simulink model "GlideslopeController_model"  (R2020b)
settings: Solver=VariableStepAuto  StartTime=0.0  StopTime=2000  RelTol=1e-3
values from neighbouring files (symbols this model uses):
  A_red_lo = sel(A_longitude_lo, [1 3 4 2 5], [1 3 4 2 5])    [GlideslopeController.m]
  B_red_lo = sel(A_longitude_lo, [1 3 4 2 5], [6 7])    [GlideslopeController.m]
  C_red_lo = sel(C_longitude_lo, [1 3 4 2 5], [1 3 4 2 5])    [GlideslopeController.m]
  D_red_lo = sel(C_longitude_lo, [1 3 4 2 5], [6 7])    [GlideslopeController.m]
  Kglide = 50    [GlideslopeController.m]
  Kq = -1    [GlideslopeController.m]
  Ktheta = 2    [GlideslopeController.m]
  Kv = 500    [GlideslopeController.m]
undefined symbols (not defined in the file or in its folder): magnitude, trim_control_lo, trim_state_lo, trim_thrust_lo
libraries: simulink_extras x10, simulink x1
settings Model: Creator=viran  LastModifiedBy=viran

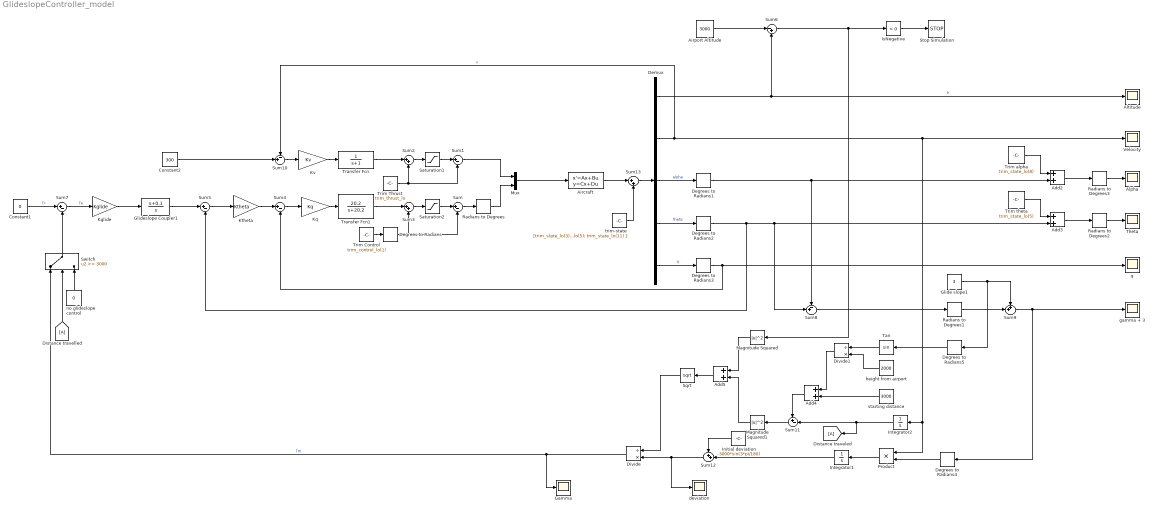
== system GlideslopeController_model ==
  " Glideslope Coupler1" : TransferFcn  Numerator=[1 0.1]  Denominator=[1 0]
  Add{2..5} (4 alike) : Sum
  Aircraft : StateSpace  A=A_red_lo  B=B_red_lo  C=C_red_lo  D=D_red_lo  InitialCondition=0
  Airport Altitude : Constant  Value=3000
  Alpha : Scope
  Altitude : Scope
  Constant1 : Constant  Value=0
  Constant2 : Constant  Value=300
  Degrees to Radians{,1..5} (6 alike) : simulink_extras/Transformations/Degrees to Radians
  Demux : Demux  Outputs=5
  Divide : Product  Inputs=/*
  Divide1 : Product  Inputs=/*
  Gamma : Scope
  Glide slope1 : Constant  Value=3
  Initial deviation : Constant  Value=-3000*sin(3*pi/180)
  Integrator1 : Integrator
  Integrator2 : Integrator
  IsNegative : simulink/Logic and Bit Operations/Compare To Zero  relop=<  OutDataTypeStr=boolean
  Kglide : Gain  Gain=Kglide
  Kq : Gain  Gain=Kq
  Ktheta : Gain  Gain=Ktheta
  Kv : Gain  Gain=Kv
  Magnitude Squared : Math  Operator=magnitude^2  SaturateOnIntegerOverflow=on
  Magnitude Squared1 : Math  Operator=magnitude^2  SaturateOnIntegerOverflow=on
  Mux : Mux  Inputs=2
  Product : Product
  Radians to Degrees{,1..3} (4 alike) : simulink_extras/Transformations/Radians to Degrees
  Saturation1 : Saturate  UpperLimit=19000  LowerLimit=1000
  Saturation2 : Saturate  UpperLimit=25*pi/180  LowerLimit=-25*pi/180
  Sqrt : Sqrt  SaturateOnIntegerOverflow=on
  Stop Simulation : Stop
  Sum{,1,4..5,7} (5 alike) : Sum  Inputs=|+-
  Sum10 : Sum  Inputs=-+|
  Sum11 : Sum  Inputs=+-|
  Sum12 : Sum  Inputs=++|
  Sum13 : Sum  Inputs=|++
  Sum2 : Sum  Inputs=|++
  Sum3 : Sum  Inputs=|++
  Sum6 : Sum  Inputs=|-+
  Sum8 : Sum  Inputs=-+|
  Sum9 : Sum  Inputs=++|
  Switch : Switch  Threshold=3000
  Tan : Trigonometry
  Theta : Scope
  Transfer Fcn : TransferFcn  Denominator=[1 1]
  Transfer Fcn1 : TransferFcn  Numerator=[20.2]  Denominator=[1 20.2]
  Trim Control : Constant  Value=trim_control_lo(1)
  Trim Thrust : Constant  Value=trim_thrust_lo
  Trim alpha : Constant  Value=trim_state_lo(8)
  Trim theta : Constant  Value=trim_state_lo(5)
  Velocity : Scope
  deviation : Scope
  gamma + 3 : Scope
  height from airport : Constant  Value=2000
  no glideslope control : Constant  Value=0
  q : Scope
  starting distance : Constant  Value=3000
  trim-state : Constant  Value=[trim_state_lo(3); trim_state_lo(7); trim_state_lo(8); trim_state_lo(5); trim_state_lo(11) ]
  wires:
  Mux/1 -> Aircraft/1
  Sum1/1 -> Mux/1
  Aircraft/1 -> Sum13/1
  Demux/3 -> Degrees to Radians1/1  "alpha"
  Demux/4 -> Degrees to Radians2/1  "theta"
  Demux/5 -> Degrees to Radians3/1  "q"
  Saturation1/1 -> Sum1/1
  Saturation2/1 -> Sum/1
  Trim Thrust/1 -> Sum1/2, Sum2/2
  Sum3/1 -> Saturation2/1
  Transfer Fcn1/1 -> Sum3/1
  Sum2/1 -> Saturation1/1
  Transfer Fcn/1 -> Sum2/1
  Trim Control/1 -> Degrees to Radians/1
  Degrees to Radians/1 -> Sum/2, Sum3/2
  Sum/1 -> Radians to Degrees/1
  Radians to Degrees/1 -> Mux/2
  Kv/1 -> Transfer Fcn/1
  Demux/1 -> Sum6/2, Altitude/1  "h"
  Demux/2 -> Sum10/1, Velocity/1, Product/1, Integrator2/1  "v"
  Sum4/1 -> Kq/1
  Kq/1 -> Transfer Fcn1/1
  Ktheta/1 -> Sum4/1
  Sum5/1 -> Ktheta/1
  " Glideslope Coupler1"/1 -> Sum5/1
  Sum10/1 -> Kv/1
  Constant2/1 -> Sum10/2
  Airport Altitude/1 -> Sum6/1
  Sum6/1 -> Magnitude Squared/1, IsNegative/1
  IsNegative/1 -> Stop Simulation/1
  Degrees to Radians1/1 -> Sum8/1, Add2/2
  Degrees to Radians2/1 -> Sum8/2, Add3/2, Sum5/2
  Add2/1 -> Radians to Degrees3/1
  Add3/1 -> Radians to Degrees2/1
  Degrees to Radians3/1 -> q/1, Sum4/2
  Trim alpha/1 -> Add2/1
  Trim theta/1 -> Add3/1
  Kglide/1 -> " Glideslope Coupler1"/1
  Sum7/1 -> Kglide/1  "Γe"
  Constant1/1 -> Sum7/1  "Γr"
  Radians to Degrees2/1 -> Theta/1
  Radians to Degrees3/1 -> Alpha/1
  Sum8/1 -> Radians to Degrees1/1
  Radians to Degrees1/1 -> Sum9/2
  Sum9/1 -> Degrees to Radians4/1, gamma + 3/1
  Glide slope1/1 -> Degrees to Radians5/1, Sum9/1
  Degrees to Radians4/1 -> Product/2
  Product/1 -> Integrator1/1
  Integrator1/1 -> Sum12/2
  no glideslope control/1 -> Switch/3
  Integrator2/1 -> [A], Sum11/2
  Sum11/1 -> Magnitude Squared1/1
  Degrees to Radians5/1 -> Tan/1
  height from airport/1 -> Divide1/2
  Tan/1 -> Divide1/1
  Add4/1 -> Sum11/1
  Divide1/1 -> Add4/1
  starting distance/1 -> Add4/2
  Magnitude Squared/1 -> Add5/1
  Magnitude Squared1/1 -> Add5/2
  Add5/1 -> Sqrt/1
  Sqrt/1 -> Divide/1
  Divide/1 -> Switch/1, Gamma/1  "Γm"
  Sum12/1 -> deviation/1, Divide/2
  Initial deviation/1 -> Sum12/1
  Sum13/1 -> Demux/1
  trim-state/1 -> Sum13/2
  Switch/1 -> Sum7/2
  [A] -> Switch/2
